simulink model "Sistema"  (R2023a)
settings: Solver=VariableStepAuto  StartTime=0.0  StopTime=10  MaxStep=1E-3  RelTol=1e-3
libraries: fl_lib x14, nesl_utility x6, slpidlib x1
settings Model: LastModifiedBy=vania
settings DataIOCC: SaveFormat=Array  ReturnWorkspaceOutputs=off  TimeSaveName=t
settings DebuggingCC: AlgebraicLoopMsg=none  ArtificialAlgebraicLoopMsg=none  MaxConsecutiveZCsMsg=none  ModelReferenceExtraNoncontSigs=none  OperatingPointInterfaceChecksumMismatchMsg=none
settings RTWCC: GPUComputeCapability=5.0

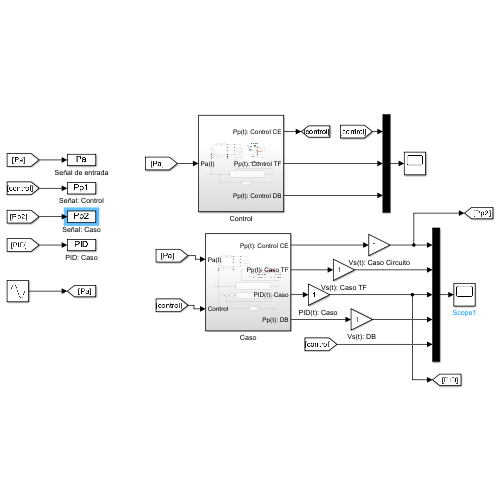
[thumbnail: Simulink's stored preview of the top-level diagram]
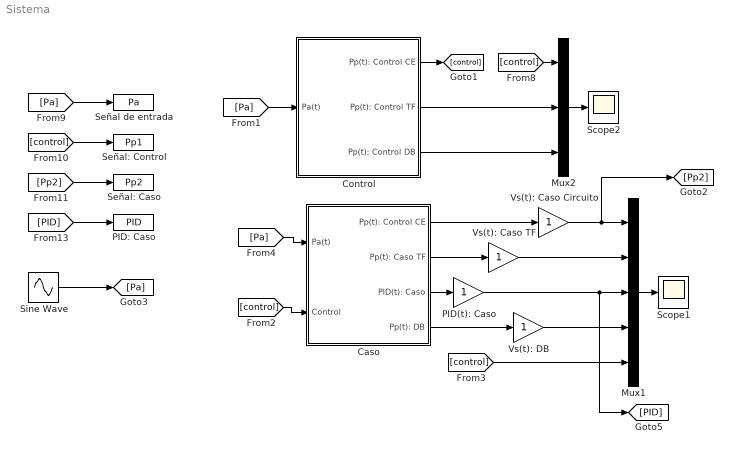
== system Sistema ==
  Caso : Subsystem
  Control : Subsystem
  Mux1 : Mux  Inputs=5
  Mux2 : Mux  Inputs=3
  "PID(t): Caso " : Gain
  PID: Caso : ToWorkspace  VariableName=PID  SampleTime=-1
  Scope1 : Scope
  Scope2 : Scope
  Señal de entrada : ToWorkspace  VariableName=Pa  SampleTime=-1
  Señal: Caso : ToWorkspace  VariableName=Pp2  SampleTime=-1
  Señal: Control : ToWorkspace  VariableName=Pp1  SampleTime=-1
  Sine Wave : Sin  Frequency=pi/2  SampleTime=0
  Vs(t): Caso Circuito : Gain
  Vs(t): Caso TF : Gain
  Vs(t): DB : Gain
  wires:
  Mux2/1 -> Scope2/1
  [Pa] -> Control/1(Pa(t))
  [Pa] -> Señal de entrada/1
  [control] -> Señal: Control/1
  [Pp2] -> Señal: Caso/1
  [PID] -> PID: Caso/1
  Mux1/1 -> Scope1/1
  [control] -> Caso/2(Control)
  Caso/1(Pp(t): Control CE) -> Vs(t): Caso Circuito/1
  [Pa] -> Caso/1(Pa(t))
  Sine Wave/1 -> [Pa]
  Control/1(Pp(t): Control CE) -> [control]
  [control] -> Mux2/1
  Control/3(Pp(t): Control DB) -> Mux2/3
  Control/2(Pp(t): Control TF) -> Mux2/2
  Vs(t): Caso Circuito/1 -> [Pp2], Mux1/1
  Caso/2(Pp(t): Caso TF) -> Vs(t): Caso TF/1
  Vs(t): Caso TF/1 -> Mux1/2
  Caso/4(Pp(t): DB) -> Vs(t): DB/1
  [control] -> Mux1/5
  Vs(t): DB/1 -> Mux1/4
  "PID(t): Caso "/1 -> Mux1/3, [PID]
  Caso/3(PID(t): Caso) -> "PID(t): Caso "/1

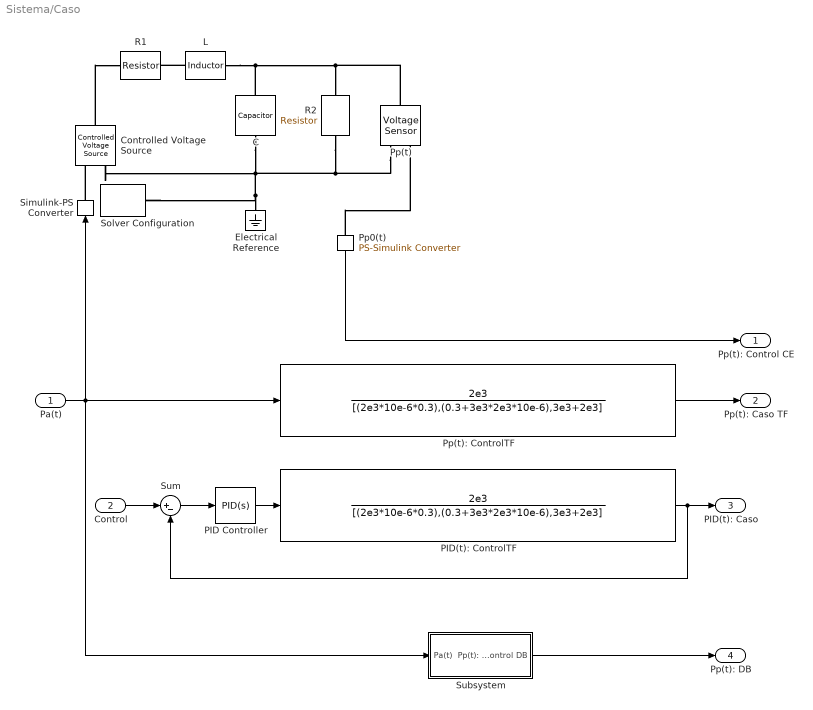
== system Sistema/Caso ==
  Pa(t) : Inport
  Control : Inport  Port=2
  C : fl_lib/Electrical/Electrical Elements/Capacitor  c=10 uF  r=1e-6 Ohm  g=0 1/Ohm  i_specify=off  i_priority=None  i=0 A  i_nominal_specify=off  i_nominal_unit=A  i_nominal_value=1  v_specify=off  v_priority=None  v=0 V  v_nominal_specify=off  v_nominal_unit=V  v_nominal_value=1  vc_specify=off  vc_priority=High  vc=0 V  vc_nominal_specify=off  vc_nominal_unit=V  vc_nominal_value=1
  Controlled Voltage Source : fl_lib/Electrical/Electrical Sources/Controlled Voltage Source
  Electrical Reference : fl_lib/Electrical/Electrical Elements/Electrical Reference
  L : fl_lib/Electrical/Electrical Elements/Inductor  l=300 mH  r=0 Ohm  g=1e-9 1/Ohm  i_specify=off  i_priority=None  i=0 A  i_nominal_specify=off  i_nominal_unit=A  i_nominal_value=1  v_specify=off  v_priority=None  v=0 V  v_nominal_specify=off  v_nominal_unit=V  v_nominal_value=1  i_L_specify=off  i_L_priority=High  i_L=0 A  i_L_nominal_specify=off  i_L_nominal_unit=A  i_L_nominal_value=1
  PID Controller : slpidlib/PID Controller  Controller=PID  Form=Parallel  TimeDomain=Continuous-time  UseExternalTs=off  SampleTime=-1  IntegratorMethod=Forward Euler  FilterMethod=Forward Euler  ControllerParametersSource=internal  P=30.3114976334533  I=8322.60743282108  UseKiTs=off  D=0.00888649215812848  N=3009.32418496381  UseFilter=on  TunerSelectOption=Transfer Function Based (PID Tuner App)  InitialConditionSource=internal  InitialConditionForIntegrator=0  InitialConditionForFilter=0  DifferentiatorICPrevScaledInput=0  ExternalReset=none  TrackingMode=off  Kt=1  LimitOutput=off  SatLimitsSource=internal  UpperSaturationLimit=inf  LowerSaturationLimit=-inf  LinearizeAsGain=on  AntiWindupMode=none  Kb=1  LimitIntegrator=off  UpperIntegratorSaturationLimit=inf  LowerIntegratorSaturationLimit=-inf  POutMin=[]  POutMax=[]  IOutMin=[]  IOutMax=[]  DOutMin=[]  DOutMax=[]  NOutMin=[]  NOutMax=[]  SumOutMin=[]  SumOutMax=[]  SaturationOutMin=[]  SaturationOutMax=[]  PParamMin=[]  PParamMax=[]  IParamMin=[]  IParamMax=[]  DParamMin=[]  DParamMax=[]  NParamMin=[]  NParamMax=[]  KbParamMin=[]  KbParamMax=[]  KtParamMin=[]  KtParamMax=[]  KbOutMin=[]  KbOutMax=[]  KtOutMin=[]  KtOutMax=[]  IntegratorOutMin=[]  IntegratorOutMax=[]  FilterOutMin=[]  FilterOutMax=[]  SumI1OutMin=[]  SumI1OutMax=[]  SumI2OutMin=[]  SumI2OutMax=[]  SumI3OutMin=[]  SumI3OutMax=[]  SumI4OutMin=[]  SumI4OutMax=[]  SumDOutMin=[]  SumDOutMax=[]  DifferentiatorOutMin=[]  DifferentiatorOutMax=[]  FilterDiffOutCoefMin=[]  FilterDiffOutCoefMax=[]  ReciprocalOutMin=[]  ReciprocalOutMax=[]  SumDenOutMin=[]  SumDenOutMax=[]  SumNumOutMin=[]  SumNumOutMax=[]  DivideOutMin=[]  DivideOutMax=[]  UdiffTsProdOutMin=[]  UdiffTsProdOutMax=[]  NTsProdOutMin=[]  NTsProdOutMax=[]  UintegralTsProdOutMin=[]  UintegralTsProdOutMax=[]  UngainTsProdOutMin=[]  UngainTsProdOutMax=[]  ClampingZeroOutDataTypeStr=Inherit: Inherit via back propagation  ClampingZeroOutMin=[]  ClampingZeroOutMax=[]  FilterDenConstantOutDataTypeStr=Inherit: Inherit via back propagation  FilterDenConstantOutMin=[]  FilterDenConstantOutMax=[]  PCopyOutDataTypeStr=Inherit: Inherit via back propagation  PCopyOutMin=[]  PCopyOutMax=[]  NCopyOutDataTypeStr=Inherit: Inherit via back propagation  NCopyOutMin=[]  NCopyOutMax=[]  IntegratorContinuousStateAttributes=''  IntegratorStateMustResolveToSignalObject=off  IntegratorRTWStateStorageClass=Auto  FilterContinuousStateAttributes=''  FilterStateMustResolveToSignalObject=off  FilterRTWStateStorageClass=Auto  ParallelPVariant=InternalParameters  IdealPVariant=Disabled  IVariant=InternalParameters  DVariant=InternalParameters  IntegratorVariant=Continuous  SatVariant=Disabled  AWVariant=Passthrough  PCopyVariant=Disabled  TRVariant=Disabled  FdbkBlocksVariant=Forward  IdealPFdbkVariant=Disabled  SatFdbkVariant=Disabled  DerivativeFilterVariant=ContFilter  NVariant=InternalParameters  NCopyVariant=Disabled  FilterICVariant=InternalICsFilter  IntegratorICVariant=InternalICs  ExternalResetVariant=Disabled  TRSumVariant=Passthrough  SumFdbkVariant=Disabled  SumVariant=Sum_PID  TsampFilterVariant=InternalTs  TsampNgainVariant=Passthrough  TsampIntegralVariant=Disabled_SignalSpec  ExternalSaturationOutDataTypeStr=Inherit: Same as second input
  PID(t): ControlTF : TransferFcn  Numerator=[2e3]  Denominator=[(2e3*10e-6*0.3),(0.3+3e3*2e3*10e-6),3e3+2e3]
  Pp(t) : fl_lib/Electrical/Electrical Sensors/Voltage Sensor
  Pp(t): ControlTF : TransferFcn  Numerator=[2e3]  Denominator=[(2e3*10e-6*0.3),(0.3+3e3*2e3*10e-6),3e3+2e3]
  Pp0(t) : nesl_utility/PS-Simulink Converter  PhysicalDomain=network_engine_domain  SubClassName=ps_output  LeftPortType=input  RightPortType=output  PseudoPeriodic=off  Frequencies=[]  VectorFormat=1-D array  Unit=inherit  AffineConversion=off
  R1 : fl_lib/Electrical/Electrical Elements/Resistor  R=3e3 Ohm  i_specify=off  i_priority=None  i=0 A  i_nominal_specify=off  i_nominal_unit=A  i_nominal_value=1  v_specify=off  v_priority=None  v=0 V  v_nominal_specify=off  v_nominal_unit=V  v_nominal_value=1
  R2 : fl_lib/Electrical/Electrical Elements/Resistor  R=2e3 Ohm  i_specify=off  i_priority=None  i=0 A  i_nominal_specify=off  i_nominal_unit=A  i_nominal_value=1  v_specify=off  v_priority=None  v=0 V  v_nominal_specify=off  v_nominal_unit=V  v_nominal_value=1
  Simulink-PS Converter : nesl_utility/Simulink-PS Converter  PhysicalDomain=network_engine_domain  SubClassName=ps_input  LeftPortType=input  RightPortType=output  PseudoPeriodic=off  Frequencies=[]  NoiseDistribution=none  NoiseParameters=[]  Unit=1  AffineConversion=off  FilteringAndDerivatives=provide  SimscapeFilterOrder=1  InputFilterTimeConstant=0.001  UdotUserProvided=0
  Solver Configuration : nesl_utility/Solver Configuration  PhysicalDomain=network_engine_domain  SubClassName=solver  LeftPortType=input  RightPortType=generic  Tones=[]  Harmonics=[]  SimulateNoise=off  Profile=off  UseLocalSampling=off  EnableSwitchedLinearOptims=on  FrequencyDomain=off  UseCCode=off  RelTol=0.001  AbsTol=0.001  MinStep=1e-09  ToWorkspace=off  RevertToSquareIcSolve=off  NumHomotopyIterations=100  PhasorMode=off  PhasorModeNumHarmonics=1  ConsistencySolver=NEWTON_XTOL_AFTER_FTOL  IndexReductionMethod=DerivativeReplacement  DoDC=off  ResidualTolerance=1e-09  ConsistencyTolSource=GLOBAL  ConsistencyAbsTol=0.001  ConsistencyRelTol=0.001  ConsistencyTolFactor=0.001  UseLocalSolver=off  LocalSolverChoice=NE_BACKWARD_EULER_ADVANCER  ResolveIndetEquations=on  FunctionEvalNumThread=1  LocalSolverSampleTime=0.001  DoFixedCost=off  MaxNonlinIter=3  MaxModeIter=2  ComputeImpulses=off  ImpulseIterations=2  LinearAlgebra=auto  LinearAlgebraNumThread=0  EquationFormulation=NE_TIME_EF  DelaysMemoryBudget=1024  AutomaticFiltering=on  FilteringTimeConstant=0.001  PartitionStorageMethod=AS_NEEDED  PartitionMemoryBudget=1024  PartitionMethod=ROBUST
  Subsystem : Subsystem
  Sum : Sum  Inputs=|+-
  Pp(t): Control CE : Outport
  Pp(t): Caso TF : Outport  Port=2
  PID(t): Caso : Outport  Port=3
  Pp(t): DB : Outport  Port=4
  wires:
  Sum/1 -> PID Controller/1
  Control/1 -> Sum/1
  PID(t): ControlTF/1 -> Sum/2, PID(t): Caso/1
  Pp(t): ControlTF/1 -> Pp(t): Caso TF/1
  Pp0(t)/1 -> Pp(t): Control CE/1
  Pa(t)/1 -> Pp(t): ControlTF/1, Subsystem/1(Pa(t)), Simulink-PS Converter/1
  PID Controller/1 -> PID(t): ControlTF/1
  Subsystem/1(Pp(t): Control DB) -> Pp(t): DB/1
  connections:
  R2/LConn1 -- Pp(t)/RConn2 -- Controlled Voltage Source/RConn2 -- Solver Configuration/RConn1 -- Electrical Reference/LConn1 -- C/LConn1
  Pp(t)/LConn1 -- L/RConn1 -- C/RConn1 -- R2/RConn1
  Simulink-PS Converter/RConn1 -- Controlled Voltage Source/RConn1
  Pp0(t)/LConn1 -- Pp(t)/RConn1
  Controlled Voltage Source/LConn1 -- R1/LConn1
  L/LConn1 -- R1/RConn1

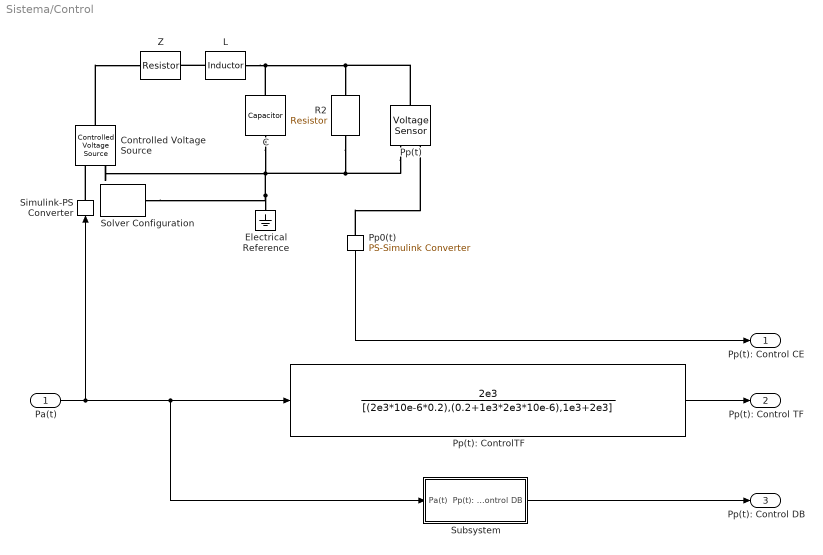
== system Sistema/Control ==
  Pa(t) : Inport
  C : fl_lib/Electrical/Electrical Elements/Capacitor  c=10 uF  r=1e-6 Ohm  g=0 1/Ohm  i_specify=off  i_priority=None  i=0 A  i_nominal_specify=off  i_nominal_unit=A  i_nominal_value=1  v_specify=off  v_priority=None  v=0 V  v_nominal_specify=off  v_nominal_unit=V  v_nominal_value=1  vc_specify=off  vc_priority=High  vc=0 V  vc_nominal_specify=off  vc_nominal_unit=V  vc_nominal_value=1
  Controlled Voltage Source : fl_lib/Electrical/Electrical Sources/Controlled Voltage Source
  Electrical Reference : fl_lib/Electrical/Electrical Elements/Electrical Reference
  L : fl_lib/Electrical/Electrical Elements/Inductor  l=200 mH  r=0 Ohm  g=1e-9 1/Ohm  i_specify=off  i_priority=None  i=0 A  i_nominal_specify=off  i_nominal_unit=A  i_nominal_value=1  v_specify=off  v_priority=None  v=0 V  v_nominal_specify=off  v_nominal_unit=V  v_nominal_value=1  i_L_specify=off  i_L_priority=High  i_L=0 A  i_L_nominal_specify=off  i_L_nominal_unit=A  i_L_nominal_value=1
  Pp(t) : fl_lib/Electrical/Electrical Sensors/Voltage Sensor
  Pp(t): ControlTF : TransferFcn  Numerator=[2e3]  Denominator=[(2e3*10e-6*0.2),(0.2+1e3*2e3*10e-6),1e3+2e3]
  Pp0(t) : nesl_utility/PS-Simulink Converter  PhysicalDomain=network_engine_domain  SubClassName=ps_output  LeftPortType=input  RightPortType=output  PseudoPeriodic=off  Frequencies=[]  VectorFormat=1-D array  Unit=inherit  AffineConversion=off
  R2 : fl_lib/Electrical/Electrical Elements/Resistor  R=2e3 Ohm  i_specify=off  i_priority=None  i=0 A  i_nominal_specify=off  i_nominal_unit=A  i_nominal_value=1  v_specify=off  v_priority=None  v=0 V  v_nominal_specify=off  v_nominal_unit=V  v_nominal_value=1
  Simulink-PS Converter : nesl_utility/Simulink-PS Converter  PhysicalDomain=network_engine_domain  SubClassName=ps_input  LeftPortType=input  RightPortType=output  PseudoPeriodic=off  Frequencies=[]  NoiseDistribution=none  NoiseParameters=[]  Unit=1  AffineConversion=off  FilteringAndDerivatives=provide  SimscapeFilterOrder=1  InputFilterTimeConstant=0.001  UdotUserProvided=0
  Solver Configuration : nesl_utility/Solver Configuration  PhysicalDomain=network_engine_domain  SubClassName=solver  LeftPortType=input  RightPortType=generic  Tones=[]  Harmonics=[]  SimulateNoise=off  Profile=off  UseLocalSampling=off  EnableSwitchedLinearOptims=on  FrequencyDomain=off  UseCCode=off  RelTol=0.001  AbsTol=0.001  MinStep=1e-09  ToWorkspace=off  RevertToSquareIcSolve=off  NumHomotopyIterations=100  PhasorMode=off  PhasorModeNumHarmonics=1  ConsistencySolver=NEWTON_XTOL_AFTER_FTOL  IndexReductionMethod=DerivativeReplacement  DoDC=off  ResidualTolerance=1e-09  ConsistencyTolSource=GLOBAL  ConsistencyAbsTol=0.001  ConsistencyRelTol=0.001  ConsistencyTolFactor=0.001  UseLocalSolver=off  LocalSolverChoice=NE_BACKWARD_EULER_ADVANCER  ResolveIndetEquations=on  FunctionEvalNumThread=1  LocalSolverSampleTime=0.001  DoFixedCost=off  MaxNonlinIter=3  MaxModeIter=2  ComputeImpulses=off  ImpulseIterations=2  LinearAlgebra=auto  LinearAlgebraNumThread=0  EquationFormulation=NE_TIME_EF  DelaysMemoryBudget=1024  AutomaticFiltering=on  FilteringTimeConstant=0.001  PartitionStorageMethod=AS_NEEDED  PartitionMemoryBudget=1024  PartitionMethod=ROBUST
  Subsystem : Subsystem
  Z : fl_lib/Electrical/Electrical Elements/Resistor  R=1e3 Ohm  i_specify=off  i_priority=None  i=0 A  i_nominal_specify=off  i_nominal_unit=A  i_nominal_value=1  v_specify=off  v_priority=None  v=0 V  v_nominal_specify=off  v_nominal_unit=V  v_nominal_value=1
  Pp(t): Control CE : Outport
  Pp(t): Control TF : Outport  Port=2
  Pp(t): Control DB : Outport  Port=3
  wires:
  Pp0(t)/1 -> Pp(t): Control CE/1
  Pp(t): ControlTF/1 -> Pp(t): Control TF/1
  Pa(t)/1 -> Subsystem/1(Pa(t)), Pp(t): ControlTF/1, Simulink-PS Converter/1
  Subsystem/1(Pp(t): Control DB) -> Pp(t): Control DB/1
  connections:
  Pp0(t)/LConn1 -- Pp(t)/RConn1
  Simulink-PS Converter/RConn1 -- Controlled Voltage Source/RConn1
  Controlled Voltage Source/RConn2 -- Pp(t)/RConn2 -- R2/LConn1 -- Solver Configuration/RConn1 -- Electrical Reference/LConn1 -- C/LConn1
  Controlled Voltage Source/LConn1 -- Z/LConn1
  Pp(t)/LConn1 -- L/RConn1 -- C/RConn1 -- R2/RConn1
  L/LConn1 -- Z/RConn1

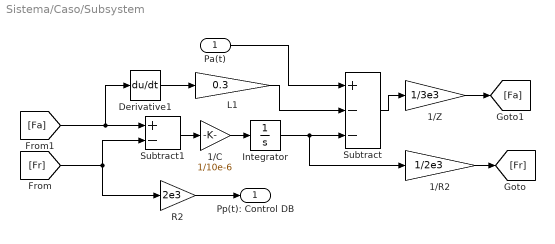
== system Sistema/Caso/Subsystem ==
  Pa(t) : Inport
  1/C : Gain  Gain=1/10e-6
  1/R2 : Gain  Gain=1/2e3
  1/Z : Gain  Gain=1/3e3
  Derivative1 : Derivative
  Integrator : Integrator
  L1 : Gain  Gain=0.3
  R2 : Gain  Gain=2e3
  Subtract : Sum  Inputs=+--
  Subtract1 : Sum  Inputs=+-
  Pp(t): Control DB : Outport
  wires:
  Derivative1/1 -> L1/1
  L1/1 -> Subtract/2
  1/Z/1 -> [Fa]
  [Fr] -> R2/1, Subtract1/2
  1/R2/1 -> [Fr]
  1/C/1 -> Integrator/1
  Subtract/1 -> 1/Z/1
  R2/1 -> Pp(t): Control DB/1
  Pa(t)/1 -> Subtract/1
  Subtract1/1 -> 1/C/1
  [Fa] -> Derivative1/1, Subtract1/1
  Integrator/1 -> 1/R2/1, Subtract/3

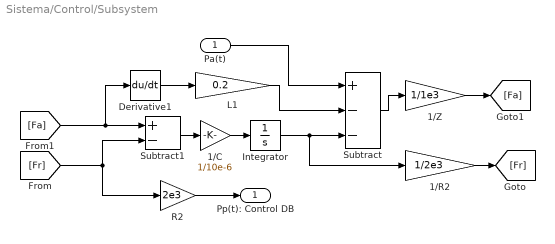
== system Sistema/Control/Subsystem ==
  Pa(t) : Inport
  1/C : Gain  Gain=1/10e-6
  1/R2 : Gain  Gain=1/2e3
  1/Z : Gain  Gain=1/1e3
  Derivative1 : Derivative
  Integrator : Integrator
  L1 : Gain  Gain=0.2
  R2 : Gain  Gain=2e3
  Subtract : Sum  Inputs=+--
  Subtract1 : Sum  Inputs=+-
  Pp(t): Control DB : Outport
  wires:
  [Fa] -> Derivative1/1, Subtract1/1
  [Fr] -> R2/1, Subtract1/2
  Subtract1/1 -> 1/C/1
  1/C/1 -> Integrator/1
  R2/1 -> Pp(t): Control DB/1
  Pa(t)/1 -> Subtract/1
  Integrator/1 -> 1/R2/1, Subtract/3
  Subtract/1 -> 1/Z/1
  1/Z/1 -> [Fa]
  1/R2/1 -> [Fr]
  L1/1 -> Subtract/2
  Derivative1/1 -> L1/1
